simulink model "BuckeyeCurrent_Simulation_2017a"  (R2017a)
settings: Solver=FixedStepAuto  StartTime=0.0  StopTime=Inf  MinStep=0.01  RelTol=1e-3
undefined symbols (not defined in the file or in its folder): A1, AIR, ambTemp_K, BATT_ELEC, BATT_OCV, BATT_THERMAL, C1, C2, COOLANT, cp, Elevation_Profile, EM, flowrate, hA1, k12, M, M2, MOT, RAD, soc0, Velocity_Profile
libraries: simulink x1
(part 2 of 2)

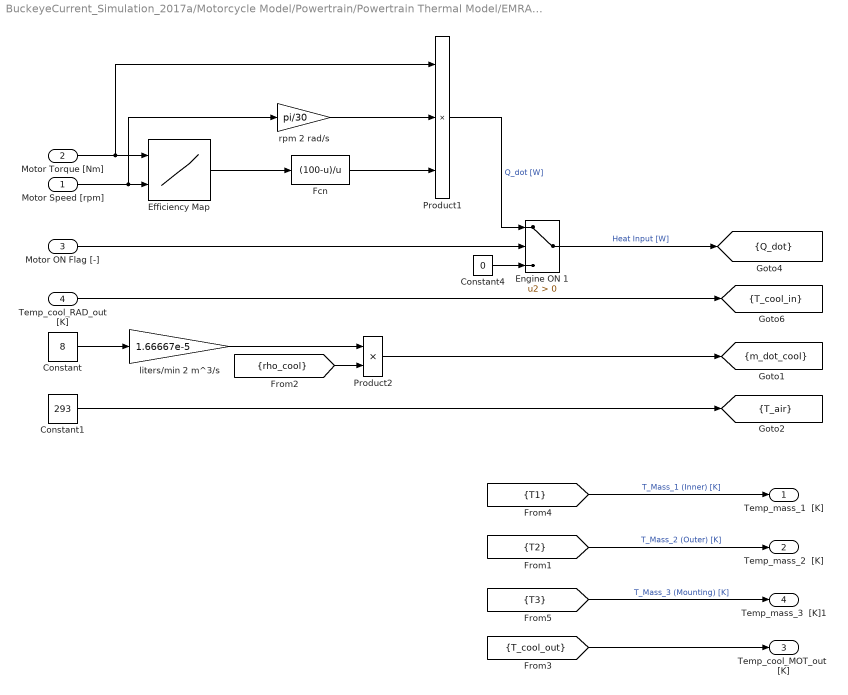
== system BuckeyeCurrent_Simulation_2017a/Motorcycle Model/Powertrain/Powertrain Thermal Model/EMRAX Motor Thermal Model/Parameter Definition ==
  Motor Speed [rpm] : Inport
  Motor Torque [Nm] : Inport  Port=2
  Motor ON Flag [-] : Inport  Port=3
  Temp_cool_RAD_out [K] : Inport  Port=4
  Constant : Constant  Value=8
  Constant1 : Constant  Value=293
  Constant4 : Constant  Value=0
  Efficiency Map : Lookup_n-D  BreakpointsForDimension1=MOT.RPM  BreakpointsForDimension2=MOT.Torque  Table=MOT.eta'  ExtrapMethod=Clip  UseLastTableValue=on  RndMeth=Simplest  InputSameDT=on
  Engine ON 1 : Switch  Criteria=u2 > Threshold
  Fcn : Fcn  Expr=(100-u)/u
  Product1 : Product  Inputs=3
  Product2 : Product
  liters/min 2 m^3/s : Gain  Gain=1.66667e-5
  rpm 2 rad/s : Gain  Gain=pi/30
  Temp_mass_1  [K] : Outport
  Temp_mass_2  [K] : Outport  Port=2
  Temp_cool_MOT_out  [K] : Outport  Port=3
  Temp_mass_3  [K]1 : Outport  Port=4
  tag scope: Q_dot=scoped, T_air=scoped, T_cool_in=scoped, m_dot_cool=scoped
  wires:
  [T1] -> Temp_mass_1  [K]/1  "T_Mass_1 (Inner) [K]"
  [T2] -> Temp_mass_2  [K]/1  "T_Mass_2 (Outer) [K]"
  Temp_cool_RAD_out [K]/1 -> [T_cool_in]
  Constant4/1 -> Engine ON 1/3
  Engine ON 1/1 -> [Q_dot]  "Heat Input [W]"
  Motor ON Flag [-]/1 -> Engine ON 1/2
  Motor Torque [Nm]/1 -> Product1/1, Efficiency Map/1
  Motor Speed [rpm]/1 -> rpm 2 rad/s/1, Efficiency Map/2
  Constant/1 -> liters/min 2 m^3/s/1
  Efficiency Map/1 -> Fcn/1
  rpm 2 rad/s/1 -> Product1/2
  Fcn/1 -> Product1/3
  Product1/1 -> Engine ON 1/1  "Q_dot [W]"
  liters/min 2 m^3/s/1 -> Product2/1
  [rho_cool] -> Product2/2
  Product2/1 -> [m_dot_cool]
  Constant1/1 -> [T_air]
  [T_cool_out] -> Temp_cool_MOT_out  [K]/1
  [T3] -> Temp_mass_3  [K]1/1  "T_Mass_3 (Mounting) [K]"

== system BuckeyeCurrent_Simulation_2017a/Motorcycle Model/Powertrain/Powertrain Thermal Model/Radiator Thermal Model/Air Properties ==
  T_air_in [K] : Inport
  Constant1 : Constant  Value=353.08
  Divide2 : Product  Inputs=*/
  Specific Heat - Air : Fcn  Expr=(AIR.cpair_a + AIR.cpair_b*u + AIR.cpair_c*u^2 + AIR.cpair_d*u^3 + AIR.cpair_e*u^4)*287
  rho_air [kg/m^3] : Outport
  cp_air [J/kg-K] : Outport  Port=2
  wires:
  Constant1/1 -> Divide2/1
  T_air_in [K]/1 -> Specific Heat - Air/1, Divide2/2
  Specific Heat - Air/1 -> cp_air [J/kg-K]/1  "cpair"
  Divide2/1 -> rho_air [kg/m^3]/1

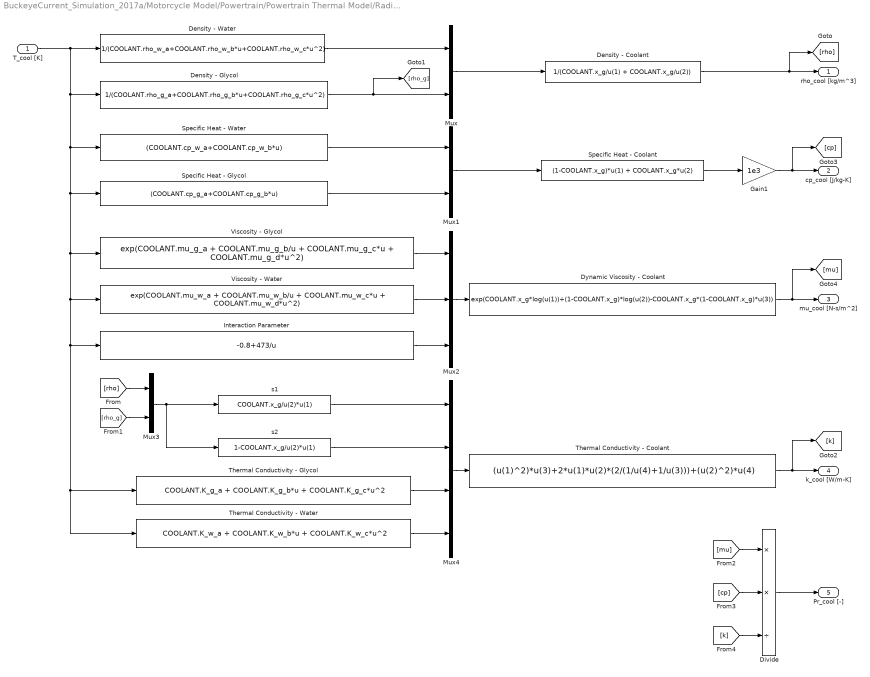
== system BuckeyeCurrent_Simulation_2017a/Motorcycle Model/Powertrain/Powertrain Thermal Model/Radiator Thermal Model/Coolant Properties ==
  T_cool [K] : Inport
  Density - Coolant : Fcn  Expr=1/(COOLANT.x_g/u(1) + COOLANT.x_g/u(2))
  Density - Glycol : Fcn  Expr=1/(COOLANT.rho_g_a+COOLANT.rho_g_b*u+COOLANT.rho_g_c*u^2)
  Density - Water : Fcn  Expr=1/(COOLANT.rho_w_a+COOLANT.rho_w_b*u+COOLANT.rho_w_c*u^2)
  Divide : Product  Inputs=**/
  Dynamic Viscosity - Coolant : Fcn  Expr=exp(COOLANT.x_g*log(u(1))+(1-COOLANT.x_g)*log(u(2))-COOLANT.x_g*(1-COOLANT.x_g)*u(3))
  Gain1 : Gain  Gain=1e3
  Interaction Parameter : Fcn  Expr=-0.8+473/u
  Mux : Mux  Inputs=2
  Mux1 : Mux  Inputs=2
  Mux2 : Mux  Inputs=3
  Mux3 : Mux  Inputs=2
  Mux4 : Mux
  Specific Heat - Coolant : Fcn  Expr=(1-COOLANT.x_g)*u(1) + COOLANT.x_g*u(2)
  Specific Heat - Glycol : Fcn  Expr=(COOLANT.cp_g_a+COOLANT.cp_g_b*u)
  Specific Heat - Water : Fcn  Expr=(COOLANT.cp_w_a+COOLANT.cp_w_b*u)
  Thermal Conductivity - Coolant : Fcn  Expr=(u(1)^2)*u(3)+2*u(1)*u(2)*(2/(1/u(4)+1/u(3)))+(u(2)^2)*u(4)
  Thermal Conductivity - Glycol : Fcn  Expr=COOLANT.K_g_a + COOLANT.K_g_b*u + COOLANT.K_g_c*u^2
  Thermal Conductivity - Water : Fcn  Expr=COOLANT.K_w_a + COOLANT.K_w_b*u + COOLANT.K_w_c*u^2
  Viscosity - Glycol : Fcn  Expr=exp(COOLANT.mu_g_a + COOLANT.mu_g_b/u + COOLANT.mu_g_c*u + COOLANT.mu_g_d*u^2)
  Viscosity - Water : Fcn  Expr=exp(COOLANT.mu_w_a + COOLANT.mu_w_b/u + COOLANT.mu_w_c*u + COOLANT.mu_w_d*u^2)
  s1 : Fcn  Expr=COOLANT.x_g/u(2)*u(1)
  s2 : Fcn  Expr=1-COOLANT.x_g/u(2)*u(1)
  rho_cool [kg/m^3] : Outport
  cp_cool [J/kg-K] : Outport  Port=2
  mu_cool [N-s/m^2] : Outport  Port=3
  k_cool [W/m-K] : Outport  Port=4
  Pr_cool [-] : Outport  Port=5
  wires:
  Density - Coolant/1 -> rho_cool [kg/m^3]/1, [rho]
  Mux/1 -> Density - Coolant/1
  T_cool [K]/1 -> Density - Water/1, Density - Glycol/1, Specific Heat - Water/1, Specific Heat - Glycol/1, Viscosity - Glycol/1, Viscosity - Water/1, Interaction Parameter/1, Thermal Conductivity - Glycol/1, Thermal Conductivity - Water/1
  Specific Heat - Coolant/1 -> Gain1/1
  Gain1/1 -> cp_cool [J/kg-K]/1, [cp]
  Mux2/1 -> Dynamic Viscosity - Coolant/1
  Viscosity - Glycol/1 -> Mux2/1
  Viscosity - Water/1 -> Mux2/2
  Interaction Parameter/1 -> Mux2/3
  Density - Water/1 -> Mux/1
  Density - Glycol/1 -> Mux/2, [rho_g]
  Dynamic Viscosity - Coolant/1 -> mu_cool [N-s/m^2]/1, [mu]
  Specific Heat - Water/1 -> Mux1/1
  Specific Heat - Glycol/1 -> Mux1/2
  Mux1/1 -> Specific Heat - Coolant/1
  Thermal Conductivity - Glycol/1 -> Mux4/3
  Thermal Conductivity - Water/1 -> Mux4/4
  Mux4/1 -> Thermal Conductivity - Coolant/1
  [rho] -> Mux3/1
  [rho_g] -> Mux3/2
  Mux3/1 -> s1/1, s2/1
  s1/1 -> Mux4/1
  s2/1 -> Mux4/2
  Thermal Conductivity - Coolant/1 -> k_cool [W/m-K]/1, [k]
  Divide/1 -> Pr_cool [-]/1
  [mu] -> Divide/1
  [cp] -> Divide/2
  [k] -> Divide/3

== system BuckeyeCurrent_Simulation_2017a/Motorcycle Model/Powertrain/Powertrain Thermal Model/Radiator Thermal Model/Reduced Radiator Thermal Model (1 Node - 1 Mass) ==
  T_cool_in [K] : Inport
  q_cool_in [m^3/s] : Inport  Port=2
  T_air [K] : Inport  Port=3
  V_face [m/s] : Inport  Port=4
  Divide3 : Product  Inputs=****
  Node 1 : Subsystem
  Sum3 : Sum  Inputs=+-
  T_cool_out [K] : Outport
  Q_dot_RAD [W] : Outport  Port=2
  wires:
  T_cool_in [K]/1 -> Node 1/1(T_c_in), Sum3/1
  T_air [K]/1 -> Node 1/3(T_air)
  Node 1/1(Tc) -> Sum3/2, T_cool_out [K]/1
  Sum3/1 -> Divide3/4
  [rho_cool] -> Divide3/1
  [cp_cool] -> Divide3/2
  Divide3/1 -> Q_dot_RAD [W]/1
  V_face [m/s]/1 -> Node 1/4(Vf)
  q_cool_in [m^3/s]/1 -> Divide3/3, Node 1/2(q_c)

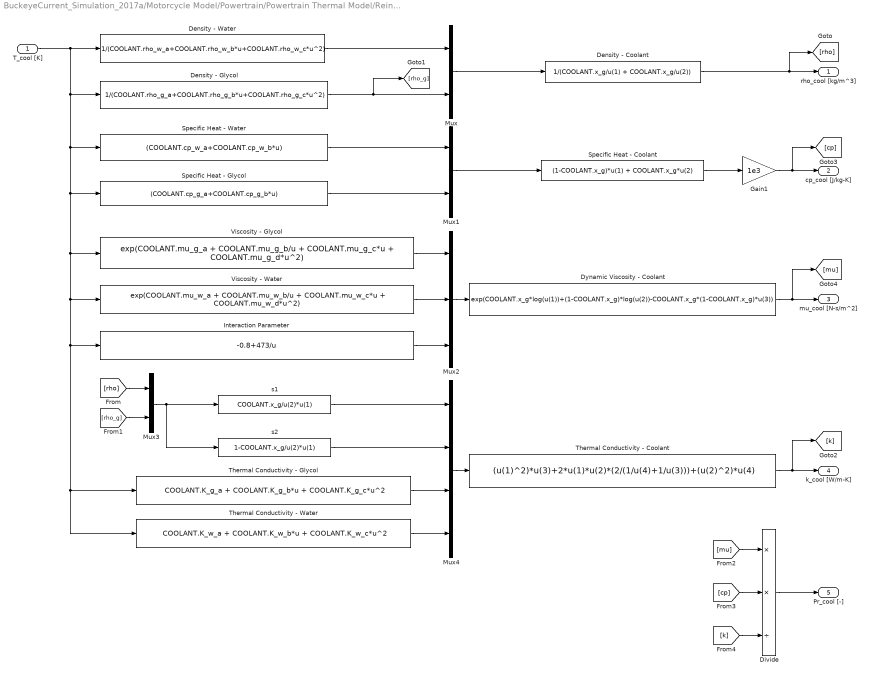
== system BuckeyeCurrent_Simulation_2017a/Motorcycle Model/Powertrain/Powertrain Thermal Model/Reinhardt Inverter Thermal Model/Coolant Properties ==
  T_cool [K] : Inport
  Density - Coolant : Fcn  Expr=1/(COOLANT.x_g/u(1) + COOLANT.x_g/u(2))
  Density - Glycol : Fcn  Expr=1/(COOLANT.rho_g_a+COOLANT.rho_g_b*u+COOLANT.rho_g_c*u^2)
  Density - Water : Fcn  Expr=1/(COOLANT.rho_w_a+COOLANT.rho_w_b*u+COOLANT.rho_w_c*u^2)
  Divide : Product  Inputs=**/
  Dynamic Viscosity - Coolant : Fcn  Expr=exp(COOLANT.x_g*log(u(1))+(1-COOLANT.x_g)*log(u(2))-COOLANT.x_g*(1-COOLANT.x_g)*u(3))
  Gain1 : Gain  Gain=1e3
  Interaction Parameter : Fcn  Expr=-0.8+473/u
  Mux : Mux  Inputs=2
  Mux1 : Mux  Inputs=2
  Mux2 : Mux  Inputs=3
  Mux3 : Mux  Inputs=2
  Mux4 : Mux
  Specific Heat - Coolant : Fcn  Expr=(1-COOLANT.x_g)*u(1) + COOLANT.x_g*u(2)
  Specific Heat - Glycol : Fcn  Expr=(COOLANT.cp_g_a+COOLANT.cp_g_b*u)
  Specific Heat - Water : Fcn  Expr=(COOLANT.cp_w_a+COOLANT.cp_w_b*u)
  Thermal Conductivity - Coolant : Fcn  Expr=(u(1)^2)*u(3)+2*u(1)*u(2)*(2/(1/u(4)+1/u(3)))+(u(2)^2)*u(4)
  Thermal Conductivity - Glycol : Fcn  Expr=COOLANT.K_g_a + COOLANT.K_g_b*u + COOLANT.K_g_c*u^2
  Thermal Conductivity - Water : Fcn  Expr=COOLANT.K_w_a + COOLANT.K_w_b*u + COOLANT.K_w_c*u^2
  Viscosity - Glycol : Fcn  Expr=exp(COOLANT.mu_g_a + COOLANT.mu_g_b/u + COOLANT.mu_g_c*u + COOLANT.mu_g_d*u^2)
  Viscosity - Water : Fcn  Expr=exp(COOLANT.mu_w_a + COOLANT.mu_w_b/u + COOLANT.mu_w_c*u + COOLANT.mu_w_d*u^2)
  s1 : Fcn  Expr=COOLANT.x_g/u(2)*u(1)
  s2 : Fcn  Expr=1-COOLANT.x_g/u(2)*u(1)
  rho_cool [kg/m^3] : Outport
  cp_cool [J/kg-K] : Outport  Port=2
  mu_cool [N-s/m^2] : Outport  Port=3
  k_cool [W/m-K] : Outport  Port=4
  Pr_cool [-] : Outport  Port=5
  wires:
  Density - Coolant/1 -> rho_cool [kg/m^3]/1, [rho]
  Mux/1 -> Density - Coolant/1
  T_cool [K]/1 -> Density - Water/1, Density - Glycol/1, Specific Heat - Water/1, Specific Heat - Glycol/1, Viscosity - Glycol/1, Viscosity - Water/1, Interaction Parameter/1, Thermal Conductivity - Glycol/1, Thermal Conductivity - Water/1
  Specific Heat - Coolant/1 -> Gain1/1
  Gain1/1 -> cp_cool [J/kg-K]/1, [cp]
  Mux2/1 -> Dynamic Viscosity - Coolant/1
  Viscosity - Glycol/1 -> Mux2/1
  Viscosity - Water/1 -> Mux2/2
  Interaction Parameter/1 -> Mux2/3
  Density - Water/1 -> Mux/1
  Density - Glycol/1 -> Mux/2, [rho_g]
  Dynamic Viscosity - Coolant/1 -> mu_cool [N-s/m^2]/1, [mu]
  Specific Heat - Water/1 -> Mux1/1
  Specific Heat - Glycol/1 -> Mux1/2
  Mux1/1 -> Specific Heat - Coolant/1
  Thermal Conductivity - Glycol/1 -> Mux4/3
  Thermal Conductivity - Water/1 -> Mux4/4
  Mux4/1 -> Thermal Conductivity - Coolant/1
  [rho] -> Mux3/1
  [rho_g] -> Mux3/2
  Mux3/1 -> s1/1, s2/1
  s1/1 -> Mux4/1
  s2/1 -> Mux4/2
  Thermal Conductivity - Coolant/1 -> k_cool [W/m-K]/1, [k]
  Divide/1 -> Pr_cool [-]/1
  [mu] -> Divide/1
  [cp] -> Divide/2
  [k] -> Divide/3

== system BuckeyeCurrent_Simulation_2017a/Motorcycle Model/Powertrain/Powertrain Thermal Model/Reinhardt Inverter Thermal Model/Inverter Thermal Model ==
  In1 : Inport
  In2 : Inport  Port=2
  In3 : Inport  Port=3
  Coolant Temp : Subsystem
  Heat Loss Calc (q_dot) : Fcn  Expr=0.000244*u(1)^1.072*u(2)^1.695+456.4
  Inverter Electrical Devices : Subsystem
  Module Case Temp : Subsystem
  Mux : Mux  Inputs=2
  Out1 : Outport
  Out2 : Outport  Port=2
  Out3 : Outport  Port=3
  tag scope: T_cool_in=global
  wires:
  In1/1 -> Mux/1  "Pack Voltage"
  In2/1 -> Mux/2  "RMS_Current"
  Mux/1 -> Heat Loss Calc (q_dot)/1
  Heat Loss Calc (q_dot)/1 -> Inverter Electrical Devices/1(Heat Rejection)
  Inverter Electrical Devices/1(Electrical Device Temps) -> Out1/1, Inverter Electrical Devices/2(Module Case Temp), Module Case Temp/1(Heat Rejection)  "Electrical Device Temps"
  Module Case Temp/1(Electrical Device Temps) -> Out2/1, Coolant Temp/1(Module Case Temp), Module Case Temp/2(Module Case Temp), Inverter Electrical Devices/3(In1)  "Module Case Temp"
  In3/1 -> [T_cool_in], Coolant Temp/2(Module Case Temp1), Module Case Temp/3(Module Case Temp1)  "Coolant Temp, in"
  Coolant Temp/1(Electrical Device Temps) -> Out3/1  "Coolant Temp, out"

== system BuckeyeCurrent_Simulation_2017a/Motorcycle Model/Powertrain/Powertrain Thermal Model/EMRAX Motor Thermal Model/3-Mass Motor Thermal Model/Mass 1 : Stator Block ==
  note: Energy Balance for Mass 1 (Inner Mass)
  Q_dot_heat [W] : Inport
  T2 [K] : Inport  Port=2
  T_cool_in [K] : Inport  Port=3
  m_dot_cool [kg/s] : Inport  Port=4
  Gain : Gain  Gain=1/(MOT.M1*MOT.C1)
  Gain1 : Gain  Gain=MOT.alpha
  Gain2 : Gain  Gain=MOT.UA1
  Gain5 : Gain  Gain=MOT.k12
  Integrator : Integrator  InitialCondition=MOT.T_init
  Product1 : Product  Inputs=*//
  Sum1 : Sum  Inputs=+-
  Sum2 : Sum  Inputs=+-
  Sum3 : Sum  Inputs=+--
  Sum5 : Sum
  T1 [K] : Outport
  T_cool_out : Outport  Port=2
  wires:
  Sum1/1 -> Gain5/1
  T2 [K]/1 -> Sum1/2
  Integrator/1 -> Sum1/1, Sum2/1, T1 [K]/1
  Sum3/1 -> Gain/1
  Q_dot_heat [W]/1 -> Gain1/1  "Engine Heat Rejection (W)"
  Gain/1 -> Integrator/1
  Gain1/1 -> Sum3/1
  Gain5/1 -> Sum3/2
  T_cool_in [K]/1 -> Sum5/1, Sum2/2
  Gain2/1 -> Product1/1, Sum3/3
  Sum2/1 -> Gain2/1
  [cp_cool] -> Product1/2
  m_dot_cool [kg/s]/1 -> Product1/3
  Product1/1 -> Sum5/2
  Sum5/1 -> T_cool_out/1

== system BuckeyeCurrent_Simulation_2017a/Motorcycle Model/Powertrain/Powertrain Thermal Model/EMRAX Motor Thermal Model/3-Mass Motor Thermal Model/Mass 2 :Rotor Block ==
  note: Energy Balance for Mass 2 (Rotor Mass)
  Q_dot_heat [W] : Inport
  T1 : Inport  Port=2
  T3 : Inport  Port=3
  Gain : Gain  Gain=1/(MOT.M2*MOT.C2)
  Gain1 : Gain  Gain=1-MOT.alpha
  Gain2 : Gain  Gain=MOT.UA2
  Gain3 : Gain  Gain=MOT.k23
  Gain5 : Gain  Gain=MOT.k12
  Integrator : Integrator  InitialCondition=MOT.T_init
  Sum1 : Sum  Inputs=+-
  Sum2 : Sum  Inputs=+-
  Sum3 : Sum  Inputs=++--
  Sum4 : Sum  Inputs=+-
  T2 [K] : Outport
  wires:
  Gain1/1 -> Sum3/1
  Gain/1 -> Integrator/1
  Q_dot_heat [W]/1 -> Gain1/1  "Engine Heat Rejection (W)"
  Sum3/1 -> Gain/1
  Integrator/1 -> Sum4/1, Sum1/2, Sum2/1, T2 [K]/1
  Sum1/1 -> Gain5/1
  Gain5/1 -> Sum3/2
  T1/1 -> Sum1/1
  Gain2/1 -> Sum3/3
  Sum2/1 -> Gain2/1
  [T_air] -> Sum2/2
  Sum4/1 -> Gain3/1
  T3/1 -> Sum4/2
  Gain3/1 -> Sum3/4

== system BuckeyeCurrent_Simulation_2017a/Motorcycle Model/Powertrain/Powertrain Thermal Model/EMRAX Motor Thermal Model/3-Mass Motor Thermal Model/Mass 3 : Motor Mounting ==
  note: Energy Balance for Mass 2 (Outer Mass)
  "T2 " : Inport
  Gain : Gain  Gain=1/(MOT.M3*MOT.C3)
  Gain2 : Gain  Gain=MOT.UA3
  Gain5 : Gain  Gain=MOT.k23
  Integrator : Integrator  InitialCondition=MOT.T_init
  Sum1 : Sum  Inputs=+-
  Sum2 : Sum  Inputs=+-
  Sum3 : Sum  Inputs=+-
  T3 [K] : Outport
  wires:
  Gain/1 -> Integrator/1
  Sum3/1 -> Gain/1
  Integrator/1 -> T3 [K]/1, Sum1/2, Sum2/1
  Sum1/1 -> Gain5/1
  "T2 "/1 -> Sum1/1
  Gain2/1 -> Sum3/2
  Sum2/1 -> Gain2/1
  [T_air] -> Sum2/2
  Gain5/1 -> Sum3/1

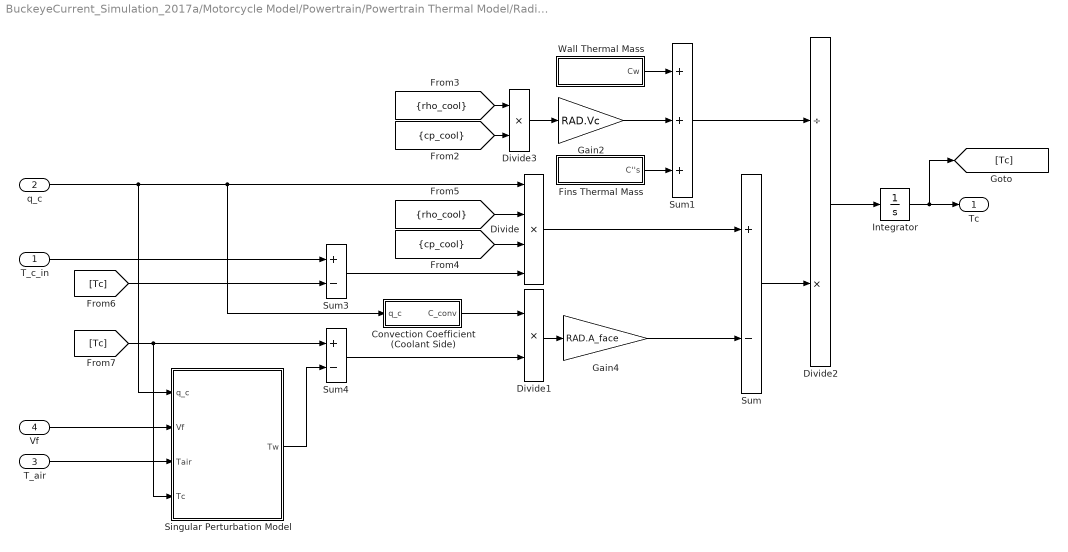
== system BuckeyeCurrent_Simulation_2017a/Motorcycle Model/Powertrain/Powertrain Thermal Model/Radiator Thermal Model/Reduced Radiator Thermal Model (1 Node - 1 Mass)/Node 1 ==
  T_c_in : Inport
  q_c : Inport  Port=2
  T_air : Inport  Port=3
  Vf : Inport  Port=4
  Convection Coefficient (Coolant Side) : Subsystem
  Divide : Product  Inputs=****
  Divide1 : Product  Inputs=**
  Divide2 : Product  Inputs=/*
  Divide3 : Product  Inputs=**
  Fins Thermal Mass : Subsystem
  Gain2 : Gain  Gain=RAD.Vc
  Gain4 : Gain  Gain=RAD.A_face
  Integrator : Integrator  InitialCondition=RAD.T_init
  Singular Perturbation Model : Subsystem
  Sum : Sum  Inputs=+-
  Sum1 : Sum  Inputs=+++
  Sum3 : Sum  Inputs=+-
  Sum4 : Sum  Inputs=+-
  Wall Thermal Mass : Subsystem
  Tc : Outport
  wires:
  Convection Coefficient (Coolant Side)/1(C_conv) -> Divide1/1
  Gain2/1 -> Sum1/2
  Wall Thermal Mass/1(Cw) -> Sum1/1
  Fins Thermal Mass/1(C''s) -> Sum1/3
  Sum1/1 -> Divide2/1
  Integrator/1 -> Tc/1, [Tc]
  [rho_cool] -> Divide3/1
  [cp_cool] -> Divide3/2
  Divide3/1 -> Gain2/1
  Divide2/1 -> Integrator/1
  Sum/1 -> Divide2/2
  q_c/1 -> Convection Coefficient (Coolant Side)/1(q_c), Divide/1, Singular Perturbation Model/1(q_c)
  [rho_cool] -> Divide/2
  [cp_cool] -> Divide/3
  Divide/1 -> Sum/1
  Sum3/1 -> Divide/4
  T_c_in/1 -> Sum3/1
  [Tc] -> Sum3/2
  Gain4/1 -> Sum/2
  Divide1/1 -> Gain4/1
  Vf/1 -> Singular Perturbation Model/2(Vf)
  Sum4/1 -> Divide1/2
  [Tc] -> Singular Perturbation Model/4(Tc), Sum4/1
  T_air/1 -> Singular Perturbation Model/3(Tair)
  Singular Perturbation Model/1(Tw) -> Sum4/2

== system BuckeyeCurrent_Simulation_2017a/Motorcycle Model/Powertrain/Powertrain Thermal Model/Reinhardt Inverter Thermal Model/Inverter Thermal Model/Coolant Temp ==
  Module Case Temp : Inport
  Module Case Temp1 : Inport  Port=2
  Gain : Gain  Gain=hA1/(flowrate*cp)
  Sum : Sum  Inputs=+-
  Sum1 : Sum  Inputs=|++
  Electrical Device Temps : Outport
  wires:
  Module Case Temp/1 -> Sum/1  "Module Case Temp"
  Sum1/1 -> Electrical Device Temps/1  "Coolant Temp, out"
  Module Case Temp1/1 -> Sum1/2, Sum/2  "Coolant Temp, in"
  Sum/1 -> Gain/1
  Gain/1 -> Sum1/1

== system BuckeyeCurrent_Simulation_2017a/Motorcycle Model/Powertrain/Powertrain Thermal Model/Reinhardt Inverter Thermal Model/Inverter Thermal Model/Inverter Electrical Devices ==
  Heat Rejection : Inport
  Module Case Temp : Inport  Port=2
  In1 : Inport  Port=3
  Gain : Gain  Gain=1/(M*C1)
  Gain1 : Gain  Gain=k12
  Integrator : Integrator
  Sum : Sum  Inputs=+-
  Sum1 : Sum  Inputs=+-
  Electrical Device Temps : Outport
  wires:
  Heat Rejection/1 -> Sum/1  "Heat Rejection"
  Module Case Temp/1 -> Sum1/1  "Electrical Device Temps"
  Integrator/1 -> Electrical Device Temps/1  "Electrical Device Temps"
  In1/1 -> Sum1/2  "Module Case Temp"
  Sum/1 -> Gain/1
  Sum1/1 -> Gain1/1
  Gain1/1 -> Sum/2
  Gain/1 -> Integrator/1  "dT1/dt"

== system BuckeyeCurrent_Simulation_2017a/Motorcycle Model/Powertrain/Powertrain Thermal Model/Reinhardt Inverter Thermal Model/Inverter Thermal Model/Module Case Temp ==
  Heat Rejection : Inport
  Module Case Temp : Inport  Port=2
  Module Case Temp1 : Inport  Port=3
  Gain1 : Gain  Gain=k12
  Gain2 : Gain  Gain=h*A1
  Gain3 : Gain  Gain=1/(M2*C2)
  Integrator : Integrator
  Sum1 : Sum  Inputs=+-
  Sum2 : Sum  Inputs=+-
  Sum3 : Sum  Inputs=+-
  Electrical Device Temps : Outport
  wires:
  Integrator/1 -> Electrical Device Temps/1  "Module Case Temp"
  Module Case Temp1/1 -> Sum2/2  "Coolant Temp, in"
  Sum1/1 -> Gain1/1
  Heat Rejection/1 -> Sum1/1  "Electrical Device Temp"
  Gain1/1 -> Sum3/1
  Module Case Temp/1 -> Sum2/1, Sum1/2  "Module Case Temp"
  Sum2/1 -> Gain2/1
  Gain2/1 -> Sum3/2
  Sum3/1 -> Gain3/1
  Gain3/1 -> Integrator/1  "dT2/dt"

== system BuckeyeCurrent_Simulation_2017a/Motorcycle Model/Powertrain/Powertrain Thermal Model/Radiator Thermal Model/Reduced Radiator Thermal Model (1 Node - 1 Mass)/Node 1/Convection Coefficient (Coolant Side) ==
  q_c : Inport
  Constant1 : Constant  Value=RAD.beta
  Constant2 : Constant  Value=1/3
  Constant3 : Constant  Value=RAD.beta
  Constant4 : Constant  Value=RAD.C3
  Divide : Product  Inputs=**/
  Divide1 : Product  Inputs=**
  Divide4 : Product  Inputs=**/
  Math Function1 : Math  Operator=pow  SaturateOnIntegerOverflow=on
  Math Function2 : Math  Operator=pow  SaturateOnIntegerOverflow=on
  Math Function3 : Math  Operator=pow  SaturateOnIntegerOverflow=on
  C_conv : Outport
  wires:
  Math Function3/1 -> Divide/3
  [mu_cool] -> Math Function3/1
  Constant3/1 -> Math Function3/2
  Math Function1/1 -> Divide/1
  Constant2/1 -> Math Function1/2
  Math Function2/1 -> Divide4/2
  Divide1/1 -> Math Function2/1
  Constant1/1 -> Math Function2/2
  [k_cool] -> Divide/2
  [Pr_cool] -> Math Function1/1
  [rho_cool] -> Divide1/1
  q_c/1 -> Divide1/2
  Constant4/1 -> Divide4/3
  Divide/1 -> Divide4/1  "Cf"
  Divide4/1 -> C_conv/1

== system BuckeyeCurrent_Simulation_2017a/Motorcycle Model/Powertrain/Powertrain Thermal Model/Radiator Thermal Model/Reduced Radiator Thermal Model (1 Node - 1 Mass)/Node 1/Fins Thermal Mass ==
  Constant1 : Constant  Value=(RAD.delt * RAD.dc * RAD.Lf) / (RAD.St * RAD.df)
  Constant2 : Constant  Value=RAD.rho_metal
  Constant4 : Constant  Value=RAD.cp_metal
  Divide4 : Product  Inputs=***
  C''s : Outport
  wires:
  Divide4/1 -> C''s/1
  Constant2/1 -> Divide4/3
  Constant4/1 -> Divide4/2
  Constant1/1 -> Divide4/1

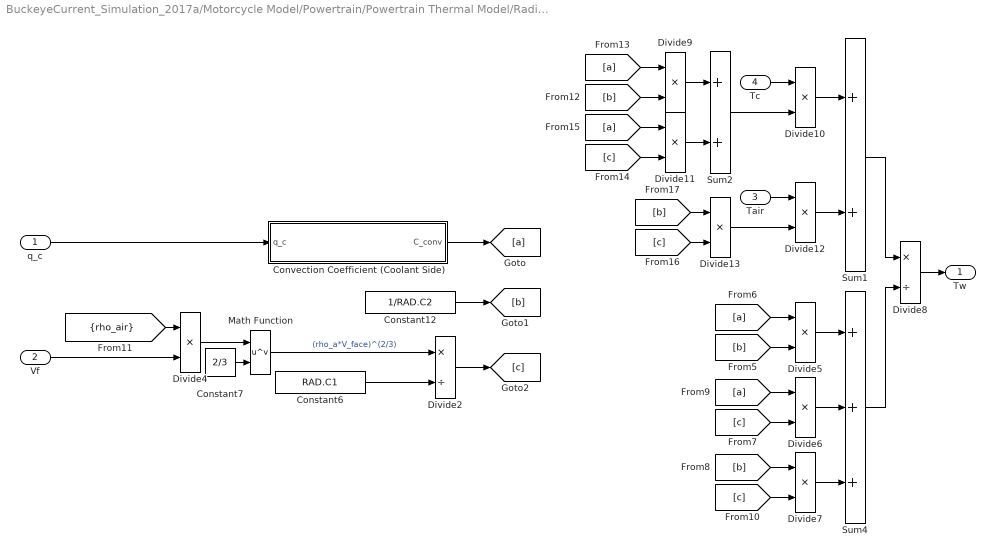
== system BuckeyeCurrent_Simulation_2017a/Motorcycle Model/Powertrain/Powertrain Thermal Model/Radiator Thermal Model/Reduced Radiator Thermal Model (1 Node - 1 Mass)/Node 1/Singular Perturbation Model ==
  q_c : Inport
  Vf : Inport  Port=2
  Tair : Inport  Port=3
  Tc : Inport  Port=4
  Constant12 : Constant  Value=1/RAD.C2
  Constant6 : Constant  Value=RAD.C1
  Constant7 : Constant  Value=2/3
  Convection Coefficient (Coolant Side) : Subsystem
  Divide{4..7,9..13} (9 alike) : Product  Inputs=**
  Divide2 : Product  Inputs=*/
  Divide8 : Product  Inputs=*/
  Math Function : Math  Operator=pow  SaturateOnIntegerOverflow=on
  Sum1 : Sum
  Sum2 : Sum
  Sum4 : Sum  Inputs=+++
  Tw : Outport
  wires:
  Divide2/1 -> [c]
  Convection Coefficient (Coolant Side)/1(C_conv) -> [a]
  Constant12/1 -> [b]
  q_c/1 -> Convection Coefficient (Coolant Side)/1(q_c)
  Sum2/1 -> Divide10/2
  Divide11/1 -> Sum2/2
  Divide9/1 -> Sum2/1
  [c] -> Divide11/2
  [a] -> Divide11/1
  Tc/1 -> Divide10/1
  Divide10/1 -> Sum1/1
  Tair/1 -> Divide12/1
  [b] -> Divide9/2
  [a] -> Divide9/1
  Divide13/1 -> Divide12/2
  [c] -> Divide13/2
  [b] -> Divide13/1
  Divide12/1 -> Sum1/2
  Sum1/1 -> Divide8/1
  Sum4/1 -> Divide8/2
  Divide7/1 -> Sum4/3
  Divide6/1 -> Sum4/2
  Divide5/1 -> Sum4/1
  [c] -> Divide7/2
  [b] -> Divide7/1
  [c] -> Divide6/2
  [a] -> Divide6/1
  [b] -> Divide5/2
  [a] -> Divide5/1
  Divide4/1 -> Math Function/1
  Constant7/1 -> Math Function/2
  Math Function/1 -> Divide2/1  "(rho_a*V_face)^(2/3)"
  Constant6/1 -> Divide2/2
  [rho_air] -> Divide4/1
  Vf/1 -> Divide4/2
  Divide8/1 -> Tw/1

== system BuckeyeCurrent_Simulation_2017a/Motorcycle Model/Powertrain/Powertrain Thermal Model/Radiator Thermal Model/Reduced Radiator Thermal Model (1 Node - 1 Mass)/Node 1/Wall Thermal Mass ==
  Constant1 : Constant  Value=RAD.St*( (RAD.dt - RAD.tt)*(RAD.tt - RAD.b) + pi/4*(RAD.dt^2 - RAD.b^2) )  VectorParams1D=off
  Constant2 : Constant  Value=RAD.rho_metal
  Constant4 : Constant  Value=RAD.cp_metal
  Divide4 : Product  Inputs=***
  Cw : Outport
  wires:
  Constant1/1 -> Divide4/1
  Constant4/1 -> Divide4/2
  Constant2/1 -> Divide4/3
  Divide4/1 -> Cw/1

== system BuckeyeCurrent_Simulation_2017a/Motorcycle Model/Powertrain/Powertrain Thermal Model/Radiator Thermal Model/Reduced Radiator Thermal Model (1 Node - 1 Mass)/Node 1/Singular Perturbation Model/Convection Coefficient (Coolant Side) ==
  q_c : Inport
  Constant1 : Constant  Value=RAD.beta
  Constant2 : Constant  Value=1/3
  Constant3 : Constant  Value=RAD.beta
  Constant4 : Constant  Value=RAD.C3
  Divide : Product  Inputs=**/
  Divide1 : Product  Inputs=**
  Divide4 : Product  Inputs=**/
  Math Function1 : Math  Operator=pow  SaturateOnIntegerOverflow=on
  Math Function2 : Math  Operator=pow  SaturateOnIntegerOverflow=on
  Math Function3 : Math  Operator=pow  SaturateOnIntegerOverflow=on
  C_conv : Outport
  wires:
  Math Function3/1 -> Divide/3
  [mu_cool] -> Math Function3/1
  Constant3/1 -> Math Function3/2
  Math Function1/1 -> Divide/1
  Constant2/1 -> Math Function1/2
  Math Function2/1 -> Divide4/2
  Divide1/1 -> Math Function2/1
  Constant1/1 -> Math Function2/2
  [k_cool] -> Divide/2
  [Pr_cool] -> Math Function1/1
  [rho_cool] -> Divide1/1
  q_c/1 -> Divide1/2
  Constant4/1 -> Divide4/3
  Divide/1 -> Divide4/1  "Cf"
  Divide4/1 -> C_conv/1
